simulink model "hinfsimapproach"  (Simulink 7.5)
settings: Solver=ode45  StartTime=0.0  StopTime=10  RelTol=1e-3
values from neighbouring files (symbols this model uses):
  A = [-0.1778 0 0 0 0 -9.7807 -9.7807 0 0 0 0 ... (first row only)    [start_h2.m]    (also in start_hinf.m; start_lqg.m)
  B = [zeros(6,4) ... (first row only)    [start_h2.m]    (also in start_hinf.m; start_lqg.m)
  C1 = C    [start_h2.m]    (also in start_hinf.m)
  D1 = D1cap    [start_h2.m]    (also in start_hinf.m)
  E = [A(:,1),A(:,2),A(:,9)]    [start_h2.m]    (also in start_hinf.m; start_lqg.m)
undefined symbols (not defined in the file or in its folder): Ao, Bo, Co
settings Model: Creator=g0800483  LastModifiedBy=A0050004
settings OptimizationCC: InitFltsAndDblsToZero=on
settings DebuggingCC: SaveWithParameterizedLinksMsg=none  MultiTaskDSMMsg=warning  MultiTaskCondExecSysMsg=none  StrictBusMsg=None
settings RTWCC: IncludeERTFirstTime=on

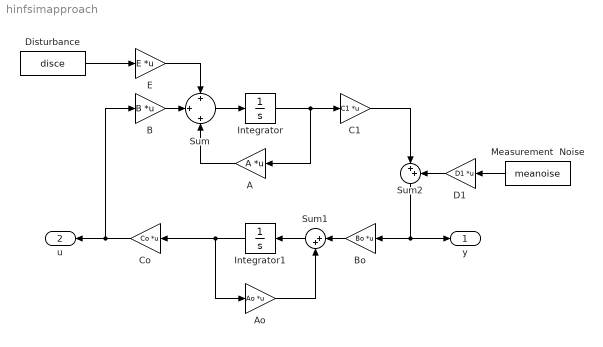
== system hinfsimapproach ==
  A : Gain  Gain=A  Multiplication=Matrix(K*u)  ParameterDataType=sfix(16)  ParameterScaling=2^0  OutDataType=sfix(16)  OutScaling=2^0
  Ao : Gain  Gain=Ao  Multiplication=Matrix(K*u)  ParameterDataType=sfix(16)  ParameterScaling=2^0  OutDataType=sfix(16)  OutScaling=2^0
  B : Gain  Gain=B  Multiplication=Matrix(K*u)  ParameterDataType=sfix(16)  ParameterScaling=2^0  OutDataType=sfix(16)  OutScaling=2^0
  Bo : Gain  Gain=Bo  Multiplication=Matrix(K*u)  ParameterDataType=sfix(16)  ParameterScaling=2^0  OutDataType=sfix(16)  OutScaling=2^0
  C1 : Gain  Gain=C1  Multiplication=Matrix(K*u)  ParameterDataType=sfix(16)  ParameterScaling=2^0  OutDataType=sfix(16)  OutScaling=2^0
  Co : Gain  Gain=Co  Multiplication=Matrix(K*u)  ParameterDataType=sfix(16)  ParameterScaling=2^0  OutDataType=sfix(16)  OutScaling=2^0
  D1 : Gain  Gain=D1  Multiplication=Matrix(K*u)  ParameterDataType=sfix(16)  ParameterScaling=2^0  OutDataType=sfix(16)  OutScaling=2^0
  Disturbance : FromWorkspace  VariableName=disce  SampleTime=0
  E : Gain  Gain=E  Multiplication=Matrix(K*u)  ParameterDataType=sfix(16)  ParameterScaling=2^0  OutDataType=sfix(16)  OutScaling=2^0
  Integrator : Integrator  InitialCondition=[1;0;0;0;0;-0.1;0;0;0;0;0]
  Integrator1 : Integrator
  Measurement  Noise : FromWorkspace  VariableName=meanoise  SampleTime=0
  Sum : Sum  Inputs=+|+|+  OutDataType=sfix(16)  OutScaling=2^0
  Sum1 : Sum  Inputs=|++  OutDataType=sfix(16)  OutScaling=2^0
  Sum2 : Sum  Inputs=|++  OutDataType=sfix(16)  OutScaling=2^0
  y : Outport  OutDataType=sfix(16)  OutScaling=2^0
  u : Outport  Port=2  OutDataType=sfix(16)  OutScaling=2^0
  wires:
  Sum/1 -> Integrator/1
  Integrator/1 -> A/1, C1/1
  Ao/1 -> Sum1/2
  Sum1/1 -> Integrator1/1
  Integrator1/1 -> Ao/1, Co/1
  C1/1 -> Sum2/1
  Sum2/1 -> y/1, Bo/1
  Co/1 -> B/1, u/1
  A/1 -> Sum/3
  B/1 -> Sum/2
  Disturbance/1 -> E/1
  E/1 -> Sum/1
  D1/1 -> Sum2/2
  Bo/1 -> Sum1/1
  Measurement  Noise/1 -> D1/1
